simulink model "L4OLARUb"  (R2020b)
settings: Solver=VariableStepAuto  StartTime=0.0  StopTime=15000  RelTol=1e-3
undefined symbols (not defined in the file or in its folder): A, B, C, D
settings Model: Creator=olaru  LastModifiedBy=olaru

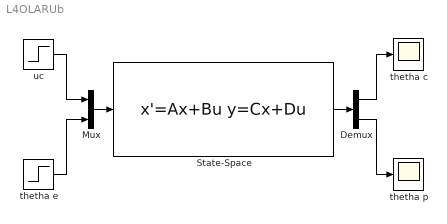
== system L4OLARUb ==
  Demux : Demux  Outputs=2
  Mux : Mux  Inputs=2
  State-Space : StateSpace  A=A  B=B  C=C  D=D  InitialCondition=0
  thetha c : Scope
  thetha e : Step  Time=5000  After=-10  SampleTime=0
  thetha p : Scope
  uc : Step  Time=0  After=2.5  SampleTime=0
  wires:
  uc/1 -> Mux/1
  thetha e/1 -> Mux/2
  Mux/1 -> State-Space/1
  State-Space/1 -> Demux/1
  Demux/1 -> thetha c/1
  Demux/2 -> thetha p/1
